simulink model "second_order"  (R2025b)
settings: Solver=VariableStepAuto  StartTime=0.0  StopTime=10.0  FixedStep=0.01  RelTol=1e-3
settings Model: Creator=Junch  LastModifiedBy=11568

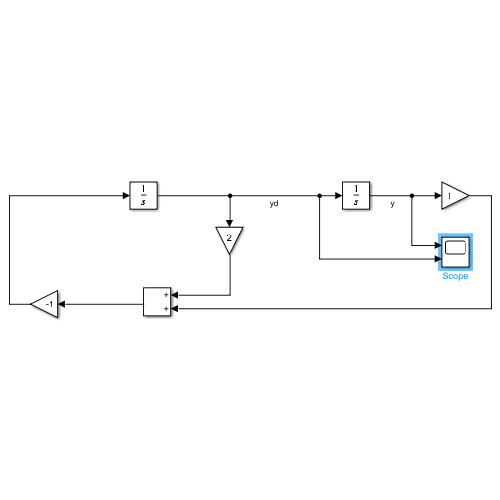
[thumbnail: Simulink's stored preview of the top-level diagram]
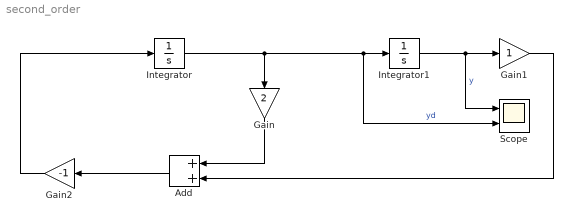
== system second_order ==
  Add : Sum
  Gain : Gain  Gain=2
  Gain1 : Gain
  Gain2 : Gain  Gain=-1
  Integrator : Integrator
  Integrator1 : Integrator  InitialCondition=1
  Scope : Scope  NumInputPorts=2
      settings: ActiveDisplayYMinimum=-0.738725936905428  ActiveDisplayYMaximum=1.1931917707672697
  wires:
  Integrator/1 -> Gain/1, Scope/2, Integrator1/1  "yd"
  Integrator1/1 -> Scope/1, Gain1/1  "y"
  Gain/1 -> Add/1
  Gain1/1 -> Add/2
  Add/1 -> Gain2/1
  Gain2/1 -> Integrator/1
